simulink model "MatlabUDPSender"  (R2018b)
settings: Solver=ode4  StartTime=0.0  StopTime=inf  FixedStep=0.1  RelTol=1e-3  EnableMultiTasking=on
libraries: commrandsrc3 x1, dspnetwork x1, instrumentlib x1
settings Model: Creator=Ssubrama  LastModifiedBy=MywinPC
settings DataIOCC: LimitDataPoints=on  SaveFormat=Array  SignalLoggingSaveFormat=ModelDataLogs
settings OptimizationCC: ExpressionDepthLimit=2147483647  InitFltsAndDblsToZero=on  LifeSpan=inf
settings DebuggingCC: UnderspecifiedInitializationDetection=Classic  MergeDetectMultiDrivingBlocksExec=none  SolverPrmCheckMsg=warning  MultiTaskDSMMsg=warning  MultiTaskCondExecSysMsg=none  FcnCallInpInsideContextMsg=warning  StateNameClashWarn=warning  SFUnexpectedBacktrackingDiag=warning  SFNoUnconditionalDefaultTransitionDiag=warning  SFExecutionAtInitializationDiag=none
settings HardwareCC: ProdBitPerPointer=32  ProdBitPerSizeT=32  ProdBitPerPtrDiffT=32  ProdLargestAtomicFloat=None  ProdIntDivRoundTo=Undefined  ProdEndianess=Unspecified  ProdWordSize=32  ProdHWDeviceType=32-bit Generic
settings ModelReferenceCC: PropagateSignalLabelsOutOfModel=off
settings SFSimCC: SimUseLocalCustomCode=off
settings RTWCC: RTWUseLocalCustomCode=off
settings CodeAppCC: StateflowObjectComments=on
settings GRTTargetCC: TargetFcnLib=ansi_tfl_tmw_new.mat  TargetLangStandard=C89/C90 (ANSI)  GeneratePreprocessorConditionals=Disable all  CombineOutputUpdateFcns=off  GRTInterface=on
settings ConfigComp: CovMetricSettings=dw  CovHtmlReporting=on  CovSaveCumulativeToWorkspaceVar=on  CovSaveSingleToWorkspaceVar=on  CovExternalEMLEnable=off

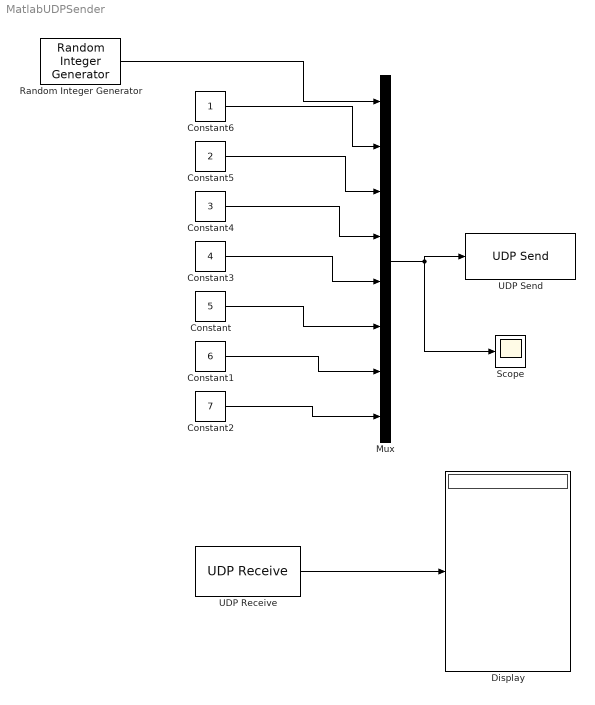
== system MatlabUDPSender ==
  Constant : Constant  Value=5  OutDataTypeStr=double
  Constant1 : Constant  Value=6  OutDataTypeStr=double
  Constant2 : Constant  Value=7  OutDataTypeStr=double
  Constant3 : Constant  Value=4  OutDataTypeStr=double
  Constant4 : Constant  Value=3  OutDataTypeStr=double
  Constant5 : Constant  Value=2  OutDataTypeStr=double
  Constant6 : Constant  OutDataTypeStr=double
  Display : Display
  Mux : Mux  Inputs=8
  Random Integer Generator : commrandsrc3/Random Integer Generator  SetSize=8  SeedSource=Parameter  Seed=1000  SampleTime=1  SamplesPerFrame=1  OutputDataType=double  SimulateUsing=Interpreted execution
  Scope : Scope
  UDP Receive : dspnetwork/UDP Receive  localURL='0.0.0.0'  localPort=10005  remoteURL='0.0.0.0'  remotePort=-1  recvBufferSize=1024  dims=255  signalDatatype=double  isVarSize=on  showBlockingTime=off  blockingTime=0  sampletime=1  blockPlatform=[]
      settings: SourceProductName=DSP System Toolbox  SourceProductBaseCode=DS
  UDP Send : instrumentlib/UDP Send  Priority=2  Host=localhost  Port=12345  LocalPort=51000  EnablePortSharing=on  ByteOrder=BigEndian  OutputDatagramPacketSize=1024  EnableBlockingMode=on  LocalAddress=0.0.0.0
      settings: SourceProductName=Instrument Control Toolbox
  wires:
  Mux/1 -> UDP Send/1, Scope/1
  Constant/1 -> Mux/6
  Constant1/1 -> Mux/7
  Constant2/1 -> Mux/8
  Constant3/1 -> Mux/5
  Constant4/1 -> Mux/4
  Constant5/1 -> Mux/3
  Constant6/1 -> Mux/2
  Random Integer Generator/1 -> Mux/1
  UDP Receive/1 -> Display/1
